simulink model "prob9"  (R2020b)
settings: Solver=VariableStepAuto  StartTime=0.0  StopTime=10.0  RelTol=1e-3
settings Model: Creator=Nitin  LastModifiedBy=Nitin

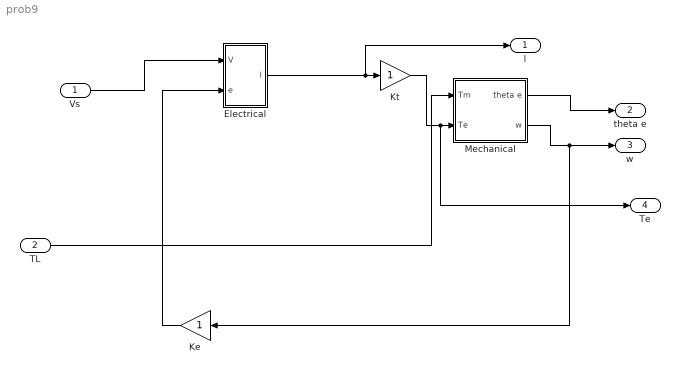
== system prob9 ==
  Vs : Inport
  TL : Inport  Port=2
  Electrical : Subsystem
  Ke : Gain
  Kt : Gain
  Mechanical : Subsystem
  l : Outport
  theta e : Outport  Port=2
  w : Outport  Port=3
  Te : Outport  Port=4
  wires:
  Vs/1 -> Electrical/1(V)
  Ke/1 -> Electrical/2(e)
  Electrical/1(l) -> Kt/1, l/1
  TL/1 -> Mechanical/1(Tm)
  Mechanical/1(theta e) -> theta e/1
  Mechanical/2(w) -> Ke/1, w/1
  Kt/1 -> Te/1, Mechanical/2(Te)

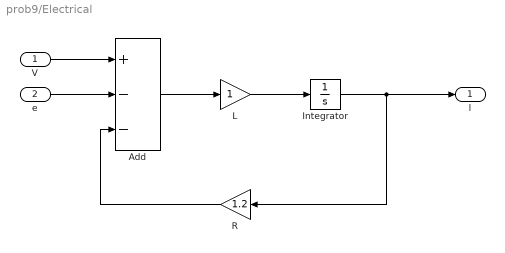
== system prob9/Electrical ==
  V : Inport
  e : Inport  Port=2
  Add : Sum  Inputs=+--
  Integrator : Integrator
  L : Gain
  R : Gain  Gain=1.2
  l : Outport
  wires:
  L/1 -> Integrator/1
  V/1 -> Add/1
  Add/1 -> L/1
  Integrator/1 -> l/1, R/1
  e/1 -> Add/2
  R/1 -> Add/3

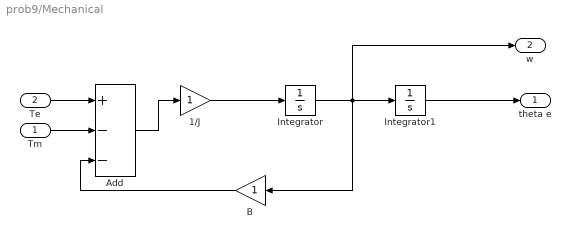
== system prob9/Mechanical ==
  Tm : Inport
  Te : Inport  Port=2
  1/J : Gain
  Add : Sum  Inputs=+--
  B : Gain
  Integrator : Integrator
  Integrator1 : Integrator
  theta e : Outport
  w : Outport  Port=2
  wires:
  Integrator1/1 -> theta e/1
  Te/1 -> Add/1
  Tm/1 -> Add/2
  Add/1 -> 1/J/1
  Integrator/1 -> w/1, B/1, Integrator1/1
  B/1 -> Add/3
  1/J/1 -> Integrator/1
